simulink model "loops"  (Simulink 7.6)
settings: Solver=FixedStepDiscrete  StartTime=0.0  StopTime=10.0  FixedStep=1  RelTol=1e-3
settings Model: Creator=ksmyth  LastModifiedBy=c2wt
settings OptimizationCC: InitFltsAndDblsToZero=on
settings DebuggingCC: SaveWithParameterizedLinksMsg=none  StrictBusMsg=Warning
settings SFSimCC: SimParseCustomCode=off
settings GRTTargetCC: TargetFcnLib=ansi_tfl_tmw.mat

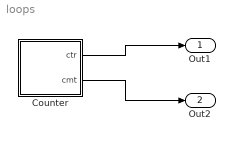
== system loops ==
  Counter : Stateflow chart  TreatAsAtomicUnit=on
  Out1 : Outport
  Out2 : Outport  Port=2
  wires:
  Counter/1(ctr) -> Out1/1
  Counter/2(cmt) -> Out2/1

== stateflow chart Counter ==
  state s1
  state group [group]
    (junction 6) -> (junction 9) : { temp = temp + 1;}
    (junction 9) -> (junction 7) [order 2] : { cmt = temp; }
    (junction 8) -> (junction 9) : { temp = -2; }
    (junction 9) -> (junction 6) [order 1] : [temp < ctr/2]
  (default) -> s1
  (junction 5) -> s1 [order 1] : [ctr < 4] / ctr = ctr+1;
  (junction 5) -> s1 [order 2] : / ctr = -2; cmt = -1;
  s1 -> (junction 8)
  (junction 7) -> (junction 5)
  data: temp local double; ctr output double =1; cmt output double
